simulink model "AC_FOC_PMSM_Developing_Rev_5_2022b"  (R2022b)
settings: Solver=VariableStepAuto  StartTime=0.0  StopTime=1  MaxStep=1e-4  RelTol=1e-3
values from neighbouring files (symbols this model uses):
  B = 11e-5    (= 0.00011)    [AB_FOC_For_PMSM_Parameters.m]
  Id_ref = 0    [AB_FOC_For_PMSM_Parameters.m]
  J = 0.47e-4    (= 4.7e-05)    [AB_FOC_For_PMSM_Parameters.m]
  Kcq = (2*zeta*wn*L) - Rs    (= 84.52)    [AB_FOC_For_PMSM_Parameters.m]
  Kcs = ((2*zeta*wns) - (B/J)) / ((1.5 *(pole^2)*flux)/J)    (= 0.00768666666667)    [AB_FOC_For_PMSM_Parameters.m]
  Ld = 7e-2    (= 0.07)    [AB_FOC_For_PMSM_Parameters.m]
  Lq = 7e-2    (= 0.07)    [AB_FOC_For_PMSM_Parameters.m]
  pole = 2    [AB_FOC_For_PMSM_Parameters.m]
  Rs = 2.98    [AB_FOC_For_PMSM_Parameters.m]
  speed_ref = 500    [AB_FOC_For_PMSM_Parameters.m]
libraries: fuzblock x10, slpidlib x9, spsDCVoltageSourceLib x5, spsPermanentMagnetSynchronousMachineLib x5, spsThreePhaseVIMeasurementLib x5, spsUniversalBridgeLib x5, spsdq0toabcLib x1, spspowerguiLib x1
(part 2 of 2)

== system AC_FOC_PMSM_Developing_Rev_5_2022b/FLC/Speed_Fuzzy_Control3 ==
  Speed_Motor : Inport
  Speed_Ref : Inport  Port=2
  Discrete PID Controller1 : slpidlib/PID Controller  Controller=I  Form=Parallel  TimeDomain=Discrete-time  UseExternalTs=off  SampleTime=-1  IntegratorMethod=Forward Euler  FilterMethod=Forward Euler  ControllerParametersSource=internal  P=1  I=0.5  UseKiTs=off  D=0  N=100  UseFilter=on  TunerSelectOption=Transfer Function Based (PID Tuner App)  InitialConditionSource=internal  InitialConditionForIntegrator=0  InitialConditionForFilter=0  DifferentiatorICPrevScaledInput=0  ExternalReset=none  TrackingMode=off  Kt=1  LimitOutput=off  SatLimitsSource=internal  UpperSaturationLimit=inf  LowerSaturationLimit=-inf  LinearizeAsGain=off  AntiWindupMode=none  Kb=1  LimitIntegrator=off  UpperIntegratorSaturationLimit=inf  LowerIntegratorSaturationLimit=-inf  POutMin=[]  POutMax=[]  IOutMin=[]  IOutMax=[]  DOutMin=[]  DOutMax=[]  NOutMin=[]  NOutMax=[]  SumOutMin=[]  SumOutMax=[]  SaturationOutMin=[]  SaturationOutMax=[]  PParamMin=[]  PParamMax=[]  IParamMin=[]  IParamMax=[]  DParamMin=[]  DParamMax=[]  NParamMin=[]  NParamMax=[]  KbParamMin=[]  KbParamMax=[]  KtParamMin=[]  KtParamMax=[]  KbOutMin=[]  KbOutMax=[]  KtOutMin=[]  KtOutMax=[]  IntegratorOutMin=[]  IntegratorOutMax=[]  FilterOutMin=[]  FilterOutMax=[]  SumI1OutMin=[]  SumI1OutMax=[]  SumI2OutMin=[]  SumI2OutMax=[]  SumI3OutMin=[]  SumI3OutMax=[]  SumI4OutMin=[]  SumI4OutMax=[]  SumDOutMin=[]  SumDOutMax=[]  DifferentiatorOutMin=[]  DifferentiatorOutMax=[]  FilterDiffOutCoefMin=[]  FilterDiffOutCoefMax=[]  ReciprocalOutMin=[]  ReciprocalOutMax=[]  SumDenOutMin=[]  SumDenOutMax=[]  SumNumOutMin=[]  SumNumOutMax=[]  DivideOutMin=[]  DivideOutMax=[]  UdiffTsProdOutMin=[]  UdiffTsProdOutMax=[]  NTsProdOutMin=[]  NTsProdOutMax=[]  UintegralTsProdOutMin=[]  UintegralTsProdOutMax=[]  UngainTsProdOutMin=[]  UngainTsProdOutMax=[]  IntegratorContinuousStateAttributes=''  IntegratorStateMustResolveToSignalObject=off  IntegratorRTWStateStorageClass=Auto  FilterContinuousStateAttributes=''  FilterStateMustResolveToSignalObject=off  FilterRTWStateStorageClass=Auto  ParallelPVariant=Disabled  IdealPVariant=Disabled  IVariant=InternalParameters  DVariant=Disabled  IntegratorVariant=Discrete  SatVariant=Disabled  AWVariant=Passthrough  PCopyVariant=Disabled  TRVariant=Disabled  FdbkBlocksVariant=Forward  IdealPFdbkVariant=Disabled  SatFdbkVariant=Disabled  DerivativeFilterVariant=Disabled  NVariant=Disabled  NCopyVariant=Disabled_SignalSpec  FilterICVariant=Disabled  IntegratorICVariant=InternalICs  ExternalResetVariant=Disabled  TRSumVariant=Passthrough  SumFdbkVariant=Disabled  SumVariant=Passthrough_I  TsampFilterVariant=InternalTs  TsampNgainVariant=Passthrough  TsampIntegralVariant=Disabled_SignalSpec  ExternalSaturationOutDataTypeStr=Inherit: Same as second input
      settings: LibrarySourceBlock=simulink/Discrete/Discrete PID Controller
  Fuzzy Logic Controller : fuzblock/Fuzzy Logic  Controller  FIS='FOC_PMSM_25_Test.fis'  OutputSampleNumber=101  DataType=double  FuzzifiedInputs=off  RuleFiringStrengths=off  RuleOutputs=off  AggregatedOutputs=off  SimulateUsing=Interpreted execution  OutOfRangeInputValueMessage=warning  NoRuleFiredMessage=warning  EmptyOutputFuzzySetMessage=warning
  Mux6 : Mux  Inputs=2
  Scope : Scope  NumInputPorts=4
  Scope1 : Scope
  Sum5 : Sum  Inputs=|+-
  Unit Delay : UnitDelay  SampleTime=-1  HasFrameUpgradeWarning=on
  Zero-Order Hold : ZeroOrderHold  SampleTime=-1
  Speed_Control : Outport
  wires:
  Mux6/1 -> Fuzzy Logic Controller/1
  Zero-Order Hold/1 -> Mux6/1, Unit Delay/1, Scope/3
  Unit Delay/1 -> Mux6/2, Scope1/1
  Speed_Motor/1 -> Scope/2, Sum5/2
  Speed_Ref/1 -> Scope/1, Sum5/1
  Fuzzy Logic Controller/1 -> Speed_Control/1
  Sum5/1 -> Zero-Order Hold/1

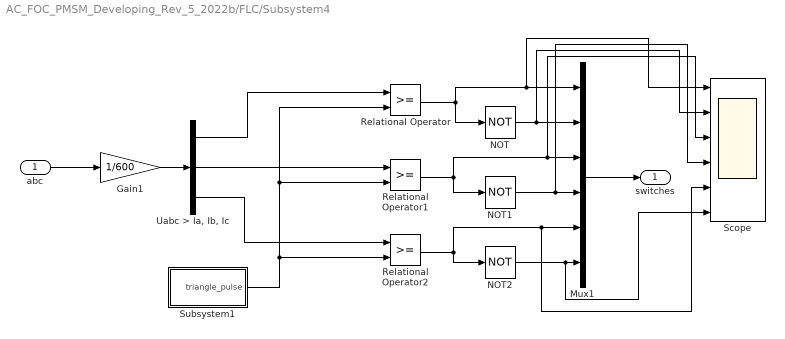
== system AC_FOC_PMSM_Developing_Rev_5_2022b/FLC/Subsystem4 ==
  abc : Inport
  Gain1 : Gain  Gain=1/600
  Mux1 : Mux  Inputs=6
  NOT : Logic  Operator=NOT  IconShape=distinctive  AllPortsSameDT=off  OutDataTypeStr=boolean
  NOT1 : Logic  Operator=NOT  IconShape=distinctive  AllPortsSameDT=off  OutDataTypeStr=boolean
  NOT2 : Logic  Operator=NOT  IconShape=distinctive  AllPortsSameDT=off  OutDataTypeStr=boolean
  Relational Operator : RelationalOperator  OutDataTypeStr=boolean  RndMeth=Simplest  InputSameDT=off
  Relational Operator1 : RelationalOperator  OutDataTypeStr=boolean  RndMeth=Simplest  InputSameDT=off
  Relational Operator2 : RelationalOperator  OutDataTypeStr=boolean  RndMeth=Simplest  InputSameDT=off
  Scope : Scope  NumInputPorts=6
  Subsystem1 : Subsystem
  "Uabc > Ia, Ib, Ic" : Demux  Outputs=3
  switches : Outport
  wires:
  NOT/1 -> Scope/2, Mux1/2
  NOT1/1 -> Scope/4, Mux1/4
  "Uabc > Ia, Ib, Ic"/2 -> Relational Operator1/1
  Gain1/1 -> "Uabc > Ia, Ib, Ic"/1
  "Uabc > Ia, Ib, Ic"/1 -> Relational Operator/1
  NOT2/1 -> Scope/6, Mux1/6
  Relational Operator1/1 -> Scope/3, Mux1/3, NOT1/1
  "Uabc > Ia, Ib, Ic"/3 -> Relational Operator2/1
  abc/1 -> Gain1/1
  Mux1/1 -> switches/1
  Relational Operator/1 -> NOT/1, Scope/1, Mux1/1
  Relational Operator2/1 -> Scope/5, Mux1/5, NOT2/1
  Subsystem1/1(triangle_pulse) -> Relational Operator/2, Relational Operator1/2, Relational Operator2/2

== system AC_FOC_PMSM_Developing_Rev_5_2022b/PID/Clark_Park Transformation ==
  Ia : Inport
  Ib : Inport  Port=2
  Ic : Inport  Port=3
  Theta : Inport  Port=4
  Gain : Gain  Gain=2/3
  Gain2 : Gain  Gain=-2/3
  Mux : Mux
  "iabc -> id" : Fcn  Expr=u(1) * sin(u(4)) + u(2) *sin(u(4) - 2*pi/3) + u(3)*sin(u(4)+2*pi/3)
  "iabc -> iq" : Fcn  Expr=u(1) * cos(u(4)) + u(2) *cos(u(4) - 2*pi/3) + u(3)*cos(u(4)+2*pi/3)
  iq : Outport
  id : Outport  Port=2
  wires:
  Gain2/1 -> id/1  "id"
  Gain/1 -> iq/1  "iq"
  "iabc -> id"/1 -> Gain2/1
  "iabc -> iq"/1 -> Gain/1
  Mux/1 -> "iabc -> iq"/1, "iabc -> id"/1
  Ia/1 -> Mux/1
  Ib/1 -> Mux/2
  Ic/1 -> Mux/3
  Theta/1 -> Mux/4

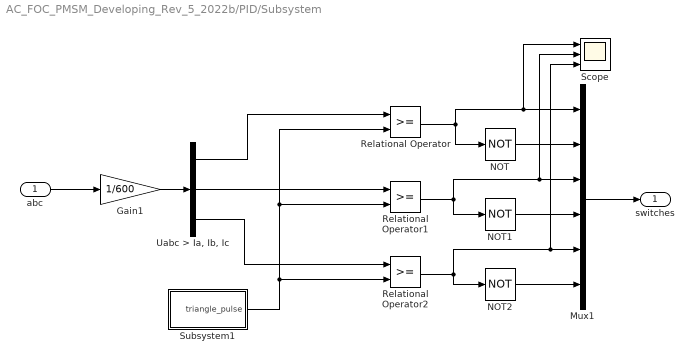
== system AC_FOC_PMSM_Developing_Rev_5_2022b/PID/Subsystem ==
  abc : Inport
  Gain1 : Gain  Gain=1/600
  Mux1 : Mux  Inputs=6
  NOT : Logic  Operator=NOT  IconShape=distinctive  AllPortsSameDT=off  OutDataTypeStr=boolean
  NOT1 : Logic  Operator=NOT  IconShape=distinctive  AllPortsSameDT=off  OutDataTypeStr=boolean
  NOT2 : Logic  Operator=NOT  IconShape=distinctive  AllPortsSameDT=off  OutDataTypeStr=boolean
  Relational Operator : RelationalOperator  OutDataTypeStr=boolean  RndMeth=Simplest  InputSameDT=off
  Relational Operator1 : RelationalOperator  OutDataTypeStr=boolean  RndMeth=Simplest  InputSameDT=off
  Relational Operator2 : RelationalOperator  OutDataTypeStr=boolean  RndMeth=Simplest  InputSameDT=off
  Scope : Scope  NumInputPorts=3
  Subsystem1 : Subsystem
  "Uabc > Ia, Ib, Ic" : Demux  Outputs=3
  switches : Outport
  wires:
  NOT/1 -> Mux1/2
  NOT1/1 -> Mux1/4
  "Uabc > Ia, Ib, Ic"/2 -> Relational Operator1/1
  Gain1/1 -> "Uabc > Ia, Ib, Ic"/1
  "Uabc > Ia, Ib, Ic"/1 -> Relational Operator/1
  NOT2/1 -> Mux1/6
  Relational Operator1/1 -> Scope/2, Mux1/3, NOT1/1
  "Uabc > Ia, Ib, Ic"/3 -> Relational Operator2/1
  abc/1 -> Gain1/1
  Mux1/1 -> switches/1
  Relational Operator/1 -> NOT/1, Scope/1, Mux1/1
  Relational Operator2/1 -> Scope/3, Mux1/5, NOT2/1
  Subsystem1/1(triangle_pulse) -> Relational Operator/2, Relational Operator1/2, Relational Operator2/2

== system AC_FOC_PMSM_Developing_Rev_5_2022b/Simplified_FLC/Clark_Park Transformation4 ==
  Ia : Inport
  Ib : Inport  Port=2
  Ic : Inport  Port=3
  Theta : Inport  Port=4
  Gain : Gain  Gain=2/3
  Gain2 : Gain  Gain=-2/3
  Mux : Mux
  "iabc -> id" : Fcn  Expr=u(1) * sin(u(4)) + u(2) *sin(u(4) - 2*pi/3) + u(3)*sin(u(4)+2*pi/3)
  "iabc -> iq" : Fcn  Expr=u(1) * cos(u(4)) + u(2) *cos(u(4) - 2*pi/3) + u(3)*cos(u(4)+2*pi/3)
  iq : Outport
  id : Outport  Port=2
  wires:
  Gain2/1 -> id/1  "id"
  Gain/1 -> iq/1  "iq"
  "iabc -> id"/1 -> Gain2/1
  "iabc -> iq"/1 -> Gain/1
  Mux/1 -> "iabc -> iq"/1, "iabc -> id"/1
  Ia/1 -> Mux/1
  Ib/1 -> Mux/2
  Ic/1 -> Mux/3
  Theta/1 -> Mux/4

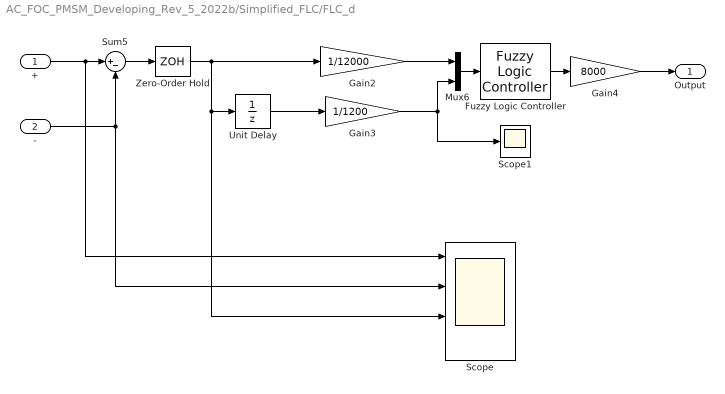
== system AC_FOC_PMSM_Developing_Rev_5_2022b/Simplified_FLC/FLC_d ==
  + : Inport
  - : Inport  Port=2
  Fuzzy Logic Controller : fuzblock/Fuzzy Logic  Controller  FIS='FOC_PMSM_25_Simplified.fis'  OutputSampleNumber=101  DataType=double  FuzzifiedInputs=off  RuleFiringStrengths=off  RuleOutputs=off  AggregatedOutputs=off  SimulateUsing=Interpreted execution  OutOfRangeInputValueMessage=warning  NoRuleFiredMessage=warning  EmptyOutputFuzzySetMessage=warning
  Gain2 : Gain  Gain=1/12000
  Gain3 : Gain  Gain=1/1200
  Gain4 : Gain  Gain=8000
  Mux6 : Mux  Inputs=2
  Scope : Scope  NumInputPorts=4
  Scope1 : Scope
  Sum5 : Sum  Inputs=|+-
  Unit Delay : UnitDelay  SampleTime=-1  HasFrameUpgradeWarning=on
  Zero-Order Hold : ZeroOrderHold  SampleTime=-1
  Output : Outport
  wires:
  Fuzzy Logic Controller/1 -> Gain4/1
  Mux6/1 -> Fuzzy Logic Controller/1
  Gain2/1 -> Mux6/1
  Gain3/1 -> Scope1/1, Mux6/2
  Gain4/1 -> Output/1
  Sum5/1 -> Zero-Order Hold/1
  -/1 -> Scope/2, Sum5/2
  +/1 -> Scope/1, Sum5/1
  Zero-Order Hold/1 -> Gain2/1, Scope/3, Unit Delay/1
  Unit Delay/1 -> Gain3/1

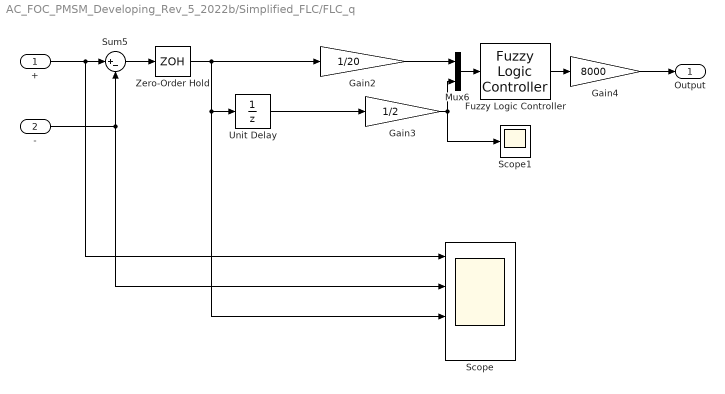
== system AC_FOC_PMSM_Developing_Rev_5_2022b/Simplified_FLC/FLC_q ==
  + : Inport
  - : Inport  Port=2
  Fuzzy Logic Controller : fuzblock/Fuzzy Logic  Controller  FIS='FOC_PMSM_25_Simplified.fis'  OutputSampleNumber=101  DataType=double  FuzzifiedInputs=off  RuleFiringStrengths=off  RuleOutputs=off  AggregatedOutputs=off  SimulateUsing=Interpreted execution  OutOfRangeInputValueMessage=warning  NoRuleFiredMessage=warning  EmptyOutputFuzzySetMessage=warning
  Gain2 : Gain  Gain=1/20
  Gain3 : Gain  Gain=1/2
  Gain4 : Gain  Gain=8000
  Mux6 : Mux  Inputs=2
  Scope : Scope  NumInputPorts=4
  Scope1 : Scope
  Sum5 : Sum  Inputs=|+-
  Unit Delay : UnitDelay  SampleTime=-1  HasFrameUpgradeWarning=on
  Zero-Order Hold : ZeroOrderHold  SampleTime=-1
  Output : Outport
  wires:
  Fuzzy Logic Controller/1 -> Gain4/1
  Mux6/1 -> Fuzzy Logic Controller/1
  Gain2/1 -> Mux6/1
  Gain3/1 -> Mux6/2, Scope1/1
  Gain4/1 -> Output/1
  Sum5/1 -> Zero-Order Hold/1
  -/1 -> Scope/2, Sum5/2
  +/1 -> Scope/1, Sum5/1
  Zero-Order Hold/1 -> Gain2/1, Scope/3, Unit Delay/1
  Unit Delay/1 -> Gain3/1

== system AC_FOC_PMSM_Developing_Rev_5_2022b/Simplified_FLC/Inverse Park-Clarke3 ==
  Iq : Inport
  Id : Inport  Port=2
  theta : Inport  Port=3
  Inverse Clarke : Subsystem
  Inverse Park : Subsystem
  Mux3 : Mux  Inputs=3
  abc : Outport
  wires:
  Inverse Park/1(alpha) -> Inverse Clarke/1(alpha)
  Inverse Clarke/2(b) -> Mux3/2
  Inverse Park/2(beta) -> Inverse Clarke/2(beta)
  Mux3/1 -> abc/1
  Inverse Clarke/1(a) -> Mux3/1
  theta/1 -> Inverse Park/3(theta)
  Iq/1 -> Inverse Park/2(Iq)
  Inverse Clarke/3(c) -> Mux3/3
  Id/1 -> Inverse Park/1(Id)

== system AC_FOC_PMSM_Developing_Rev_5_2022b/Simplified_FLC/Speed_Fuzzy_Control3 ==
  Speed_Motor : Inport
  Speed_Ref : Inport  Port=2
  Fuzzy Logic Controller : fuzblock/Fuzzy Logic  Controller  FIS='FOC_PMSM_25_Simplified.fis'  OutputSampleNumber=101  DataType=double  FuzzifiedInputs=off  RuleFiringStrengths=off  RuleOutputs=off  AggregatedOutputs=off  SimulateUsing=Interpreted execution  OutOfRangeInputValueMessage=warning  NoRuleFiredMessage=warning  EmptyOutputFuzzySetMessage=warning
  Gain2 : Gain  Gain=1/2500
  Gain3 : Gain  Gain=1/2500
  Gain4 : Gain  Gain=50
  Mux6 : Mux  Inputs=2
  Scope : Scope  NumInputPorts=4
  Scope1 : Scope
  Sum5 : Sum  Inputs=|+-
  Unit Delay : UnitDelay  SampleTime=-1  HasFrameUpgradeWarning=on
  Zero-Order Hold : ZeroOrderHold  SampleTime=-1
  Speed_Control : Outport
  wires:
  Fuzzy Logic Controller/1 -> Gain4/1
  Mux6/1 -> Fuzzy Logic Controller/1
  Gain2/1 -> Mux6/1
  Gain3/1 -> Mux6/2, Scope1/1
  Gain4/1 -> Speed_Control/1
  Sum5/1 -> Zero-Order Hold/1
  Speed_Motor/1 -> Scope/2, Sum5/2
  Speed_Ref/1 -> Scope/1, Sum5/1
  Zero-Order Hold/1 -> Gain2/1, Unit Delay/1, Scope/3
  Unit Delay/1 -> Gain3/1

== system AC_FOC_PMSM_Developing_Rev_5_2022b/Simplified_FLC/Subsystem4 ==
  abc : Inport
  Gain1 : Gain  Gain=1/600
  Mux1 : Mux  Inputs=6
  NOT : Logic  Operator=NOT  IconShape=distinctive  AllPortsSameDT=off  OutDataTypeStr=boolean
  NOT1 : Logic  Operator=NOT  IconShape=distinctive  AllPortsSameDT=off  OutDataTypeStr=boolean
  NOT2 : Logic  Operator=NOT  IconShape=distinctive  AllPortsSameDT=off  OutDataTypeStr=boolean
  Relational Operator : RelationalOperator  OutDataTypeStr=boolean  RndMeth=Simplest  InputSameDT=off
  Relational Operator1 : RelationalOperator  OutDataTypeStr=boolean  RndMeth=Simplest  InputSameDT=off
  Relational Operator2 : RelationalOperator  OutDataTypeStr=boolean  RndMeth=Simplest  InputSameDT=off
  Scope : Scope  NumInputPorts=6
  Subsystem1 : Subsystem
  "Uabc > Ia, Ib, Ic" : Demux  Outputs=3
  switches : Outport
  wires:
  NOT/1 -> Scope/2, Mux1/2
  NOT1/1 -> Scope/4, Mux1/4
  "Uabc > Ia, Ib, Ic"/2 -> Relational Operator1/1
  Gain1/1 -> "Uabc > Ia, Ib, Ic"/1
  "Uabc > Ia, Ib, Ic"/1 -> Relational Operator/1
  NOT2/1 -> Scope/6, Mux1/6
  Relational Operator1/1 -> Scope/3, Mux1/3, NOT1/1
  "Uabc > Ia, Ib, Ic"/3 -> Relational Operator2/1
  abc/1 -> Gain1/1
  Mux1/1 -> switches/1
  Relational Operator/1 -> NOT/1, Scope/1, Mux1/1
  Relational Operator2/1 -> Scope/5, Mux1/5, NOT2/1
  Subsystem1/1(triangle_pulse) -> Relational Operator/2, Relational Operator1/2, Relational Operator2/2

== system AC_FOC_PMSM_Developing_Rev_5_2022b/Simplified_Speed_Q_FLC_D_PID1/Clark_Park Transformation4 ==
  Ia : Inport
  Ib : Inport  Port=2
  Ic : Inport  Port=3
  Theta : Inport  Port=4
  Gain : Gain  Gain=2/3
  Gain2 : Gain  Gain=-2/3
  Mux : Mux
  "iabc -> id" : Fcn  Expr=u(1) * sin(u(4)) + u(2) *sin(u(4) - 2*pi/3) + u(3)*sin(u(4)+2*pi/3)
  "iabc -> iq" : Fcn  Expr=u(1) * cos(u(4)) + u(2) *cos(u(4) - 2*pi/3) + u(3)*cos(u(4)+2*pi/3)
  iq : Outport
  id : Outport  Port=2
  wires:
  Gain2/1 -> id/1  "id"
  Gain/1 -> iq/1  "iq"
  "iabc -> id"/1 -> Gain2/1
  "iabc -> iq"/1 -> Gain/1
  Mux/1 -> "iabc -> iq"/1, "iabc -> id"/1
  Ia/1 -> Mux/1
  Ib/1 -> Mux/2
  Ic/1 -> Mux/3
  Theta/1 -> Mux/4

== system AC_FOC_PMSM_Developing_Rev_5_2022b/Simplified_Speed_Q_FLC_D_PID1/FLC_q2 ==
  + : Inport
  - : Inport  Port=2
  Fuzzy Logic Controller : fuzblock/Fuzzy Logic  Controller  FIS='FOC_PMSM_25.fis'  OutputSampleNumber=101  DataType=double  FuzzifiedInputs=off  RuleFiringStrengths=off  RuleOutputs=off  AggregatedOutputs=off  SimulateUsing=Interpreted execution  OutOfRangeInputValueMessage=warning  NoRuleFiredMessage=warning  EmptyOutputFuzzySetMessage=warning
  Gain2 : Gain  Gain=1/20
  Gain3 : Gain  Gain=1/2
  Gain4 : Gain  Gain=8000
  Mux6 : Mux  Inputs=2
  Scope : Scope  NumInputPorts=4
  Scope1 : Scope
  Sum5 : Sum  Inputs=|+-
  Unit Delay : UnitDelay  SampleTime=-1  HasFrameUpgradeWarning=on
  Zero-Order Hold : ZeroOrderHold  SampleTime=-1
  Output : Outport
  wires:
  Fuzzy Logic Controller/1 -> Gain4/1
  Mux6/1 -> Fuzzy Logic Controller/1
  Gain2/1 -> Mux6/1
  Gain3/1 -> Mux6/2, Scope1/1
  Gain4/1 -> Output/1
  Sum5/1 -> Zero-Order Hold/1
  -/1 -> Scope/2, Sum5/2
  +/1 -> Scope/1, Sum5/1
  Zero-Order Hold/1 -> Gain2/1, Scope/3, Unit Delay/1
  Unit Delay/1 -> Gain3/1

== system AC_FOC_PMSM_Developing_Rev_5_2022b/Simplified_Speed_Q_FLC_D_PID1/Inverse Park-Clarke3 ==
  Iq : Inport
  Id : Inport  Port=2
  theta : Inport  Port=3
  Inverse Clarke : Subsystem
  Inverse Park : Subsystem
  Mux3 : Mux  Inputs=3
  abc : Outport
  wires:
  Inverse Park/1(alpha) -> Inverse Clarke/1(alpha)
  Inverse Clarke/2(b) -> Mux3/2
  Inverse Park/2(beta) -> Inverse Clarke/2(beta)
  Mux3/1 -> abc/1
  Inverse Clarke/1(a) -> Mux3/1
  theta/1 -> Inverse Park/3(theta)
  Iq/1 -> Inverse Park/2(Iq)
  Inverse Clarke/3(c) -> Mux3/3
  Id/1 -> Inverse Park/1(Id)

== system AC_FOC_PMSM_Developing_Rev_5_2022b/Simplified_Speed_Q_FLC_D_PID1/Speed_Fuzzy_Control3 ==
  Speed_Motor : Inport
  Speed_Ref : Inport  Port=2
  Fuzzy Logic Controller : fuzblock/Fuzzy Logic  Controller  FIS='FOC_PMSM_25_Simplified.fis'  OutputSampleNumber=101  DataType=double  FuzzifiedInputs=off  RuleFiringStrengths=off  RuleOutputs=off  AggregatedOutputs=off  SimulateUsing=Interpreted execution  OutOfRangeInputValueMessage=warning  NoRuleFiredMessage=warning  EmptyOutputFuzzySetMessage=warning
  Gain2 : Gain  Gain=1/2500
  Gain3 : Gain  Gain=1/2500
  Gain4 : Gain  Gain=50
  Mux6 : Mux  Inputs=2
  Scope : Scope  NumInputPorts=4
  Scope1 : Scope
  Sum5 : Sum  Inputs=|+-
  Unit Delay : UnitDelay  SampleTime=-1  HasFrameUpgradeWarning=on
  Zero-Order Hold : ZeroOrderHold  SampleTime=-1
  Speed_Control : Outport
  wires:
  Fuzzy Logic Controller/1 -> Gain4/1
  Mux6/1 -> Fuzzy Logic Controller/1
  Gain2/1 -> Mux6/1
  Gain3/1 -> Mux6/2, Scope1/1
  Gain4/1 -> Speed_Control/1
  Sum5/1 -> Zero-Order Hold/1
  Speed_Motor/1 -> Scope/2, Sum5/2
  Speed_Ref/1 -> Scope/1, Sum5/1
  Zero-Order Hold/1 -> Gain2/1, Unit Delay/1, Scope/3
  Unit Delay/1 -> Gain3/1

== system AC_FOC_PMSM_Developing_Rev_5_2022b/Simplified_Speed_Q_FLC_D_PID1/Subsystem4 ==
  abc : Inport
  Gain1 : Gain  Gain=1/600
  Mux1 : Mux  Inputs=6
  NOT : Logic  Operator=NOT  IconShape=distinctive  AllPortsSameDT=off  OutDataTypeStr=boolean
  NOT1 : Logic  Operator=NOT  IconShape=distinctive  AllPortsSameDT=off  OutDataTypeStr=boolean
  NOT2 : Logic  Operator=NOT  IconShape=distinctive  AllPortsSameDT=off  OutDataTypeStr=boolean
  Relational Operator : RelationalOperator  OutDataTypeStr=boolean  RndMeth=Simplest  InputSameDT=off
  Relational Operator1 : RelationalOperator  OutDataTypeStr=boolean  RndMeth=Simplest  InputSameDT=off
  Relational Operator2 : RelationalOperator  OutDataTypeStr=boolean  RndMeth=Simplest  InputSameDT=off
  Scope : Scope  NumInputPorts=6
  Subsystem1 : Subsystem
  "Uabc > Ia, Ib, Ic" : Demux  Outputs=3
  switches : Outport
  wires:
  NOT/1 -> Scope/2, Mux1/2
  NOT1/1 -> Scope/4, Mux1/4
  "Uabc > Ia, Ib, Ic"/2 -> Relational Operator1/1
  Gain1/1 -> "Uabc > Ia, Ib, Ic"/1
  "Uabc > Ia, Ib, Ic"/1 -> Relational Operator/1
  NOT2/1 -> Scope/6, Mux1/6
  Relational Operator1/1 -> Scope/3, Mux1/3, NOT1/1
  "Uabc > Ia, Ib, Ic"/3 -> Relational Operator2/1
  abc/1 -> Gain1/1
  Mux1/1 -> switches/1
  Relational Operator/1 -> NOT/1, Scope/1, Mux1/1
  Relational Operator2/1 -> Scope/5, Mux1/5, NOT2/1
  Subsystem1/1(triangle_pulse) -> Relational Operator/2, Relational Operator1/2, Relational Operator2/2

== system AC_FOC_PMSM_Developing_Rev_5_2022b/Speed_Q_FLC_D_PID/Clark_Park Transformation4 ==
  Ia : Inport
  Ib : Inport  Port=2
  Ic : Inport  Port=3
  Theta : Inport  Port=4
  Gain : Gain  Gain=2/3
  Gain2 : Gain  Gain=-2/3
  Mux : Mux
  "iabc -> id" : Fcn  Expr=u(1) * sin(u(4)) + u(2) *sin(u(4) - 2*pi/3) + u(3)*sin(u(4)+2*pi/3)
  "iabc -> iq" : Fcn  Expr=u(1) * cos(u(4)) + u(2) *cos(u(4) - 2*pi/3) + u(3)*cos(u(4)+2*pi/3)
  iq : Outport
  id : Outport  Port=2
  wires:
  Gain2/1 -> id/1  "id"
  Gain/1 -> iq/1  "iq"
  "iabc -> id"/1 -> Gain2/1
  "iabc -> iq"/1 -> Gain/1
  Mux/1 -> "iabc -> iq"/1, "iabc -> id"/1
  Ia/1 -> Mux/1
  Ib/1 -> Mux/2
  Ic/1 -> Mux/3
  Theta/1 -> Mux/4

== system AC_FOC_PMSM_Developing_Rev_5_2022b/Speed_Q_FLC_D_PID/FLC_q2 ==
  + : Inport
  - : Inport  Port=2
  Fuzzy Logic Controller : fuzblock/Fuzzy Logic  Controller  FIS='FOC_PMSM_25.fis'  OutputSampleNumber=101  DataType=double  FuzzifiedInputs=off  RuleFiringStrengths=off  RuleOutputs=off  AggregatedOutputs=off  SimulateUsing=Interpreted execution  OutOfRangeInputValueMessage=warning  NoRuleFiredMessage=warning  EmptyOutputFuzzySetMessage=warning
  Gain2 : Gain  Gain=1/20
  Gain3 : Gain  Gain=1/2
  Gain4 : Gain  Gain=8000
  Mux6 : Mux  Inputs=2
  Scope : Scope  NumInputPorts=4
  Scope1 : Scope
  Sum5 : Sum  Inputs=|+-
  Unit Delay : UnitDelay  SampleTime=-1  HasFrameUpgradeWarning=on
  Zero-Order Hold : ZeroOrderHold  SampleTime=-1
  Output : Outport
  wires:
  Fuzzy Logic Controller/1 -> Gain4/1
  Mux6/1 -> Fuzzy Logic Controller/1
  Gain2/1 -> Mux6/1
  Gain3/1 -> Mux6/2, Scope1/1
  Gain4/1 -> Output/1
  Sum5/1 -> Zero-Order Hold/1
  -/1 -> Scope/2, Sum5/2
  +/1 -> Scope/1, Sum5/1
  Zero-Order Hold/1 -> Gain2/1, Scope/3, Unit Delay/1
  Unit Delay/1 -> Gain3/1

== system AC_FOC_PMSM_Developing_Rev_5_2022b/Speed_Q_FLC_D_PID/Inverse Park-Clarke3 ==
  Iq : Inport
  Id : Inport  Port=2
  theta : Inport  Port=3
  Inverse Clarke : Subsystem
  Inverse Park : Subsystem
  Mux3 : Mux  Inputs=3
  abc : Outport
  wires:
  Inverse Park/1(alpha) -> Inverse Clarke/1(alpha)
  Inverse Clarke/2(b) -> Mux3/2
  Inverse Park/2(beta) -> Inverse Clarke/2(beta)
  Mux3/1 -> abc/1
  Inverse Clarke/1(a) -> Mux3/1
  theta/1 -> Inverse Park/3(theta)
  Iq/1 -> Inverse Park/2(Iq)
  Inverse Clarke/3(c) -> Mux3/3
  Id/1 -> Inverse Park/1(Id)

== system AC_FOC_PMSM_Developing_Rev_5_2022b/Speed_Q_FLC_D_PID/Speed_Fuzzy_Control3 ==
  Speed_Motor : Inport
  Speed_Ref : Inport  Port=2
  Fuzzy Logic Controller : fuzblock/Fuzzy Logic  Controller  FIS='FOC_PMSM_25.fis'  OutputSampleNumber=101  DataType=double  FuzzifiedInputs=off  RuleFiringStrengths=off  RuleOutputs=off  AggregatedOutputs=off  SimulateUsing=Interpreted execution  OutOfRangeInputValueMessage=warning  NoRuleFiredMessage=warning  EmptyOutputFuzzySetMessage=warning
  Gain2 : Gain  Gain=1/2500
  Gain3 : Gain  Gain=1/2500
  Gain4 : Gain  Gain=50
  Mux6 : Mux  Inputs=2
  Scope : Scope  NumInputPorts=4
  Scope1 : Scope
  Sum5 : Sum  Inputs=|+-
  Unit Delay : UnitDelay  SampleTime=-1  HasFrameUpgradeWarning=on
  Zero-Order Hold : ZeroOrderHold  SampleTime=-1
  Speed_Control : Outport
  wires:
  Fuzzy Logic Controller/1 -> Gain4/1
  Mux6/1 -> Fuzzy Logic Controller/1
  Gain2/1 -> Mux6/1
  Gain3/1 -> Mux6/2, Scope1/1
  Gain4/1 -> Speed_Control/1
  Sum5/1 -> Zero-Order Hold/1
  Speed_Motor/1 -> Scope/2, Sum5/2
  Speed_Ref/1 -> Scope/1, Sum5/1
  Zero-Order Hold/1 -> Gain2/1, Unit Delay/1, Scope/3
  Unit Delay/1 -> Gain3/1

== system AC_FOC_PMSM_Developing_Rev_5_2022b/Speed_Q_FLC_D_PID/Subsystem4 ==
  abc : Inport
  Gain1 : Gain  Gain=1/600
  Mux1 : Mux  Inputs=6
  NOT : Logic  Operator=NOT  IconShape=distinctive  AllPortsSameDT=off  OutDataTypeStr=boolean
  NOT1 : Logic  Operator=NOT  IconShape=distinctive  AllPortsSameDT=off  OutDataTypeStr=boolean
  NOT2 : Logic  Operator=NOT  IconShape=distinctive  AllPortsSameDT=off  OutDataTypeStr=boolean
  Relational Operator : RelationalOperator  OutDataTypeStr=boolean  RndMeth=Simplest  InputSameDT=off
  Relational Operator1 : RelationalOperator  OutDataTypeStr=boolean  RndMeth=Simplest  InputSameDT=off
  Relational Operator2 : RelationalOperator  OutDataTypeStr=boolean  RndMeth=Simplest  InputSameDT=off
  Scope : Scope  NumInputPorts=6
  Subsystem1 : Subsystem
  "Uabc > Ia, Ib, Ic" : Demux  Outputs=3
  switches : Outport
  wires:
  NOT/1 -> Scope/2, Mux1/2
  NOT1/1 -> Scope/4, Mux1/4
  "Uabc > Ia, Ib, Ic"/2 -> Relational Operator1/1
  Gain1/1 -> "Uabc > Ia, Ib, Ic"/1
  "Uabc > Ia, Ib, Ic"/1 -> Relational Operator/1
  NOT2/1 -> Scope/6, Mux1/6
  Relational Operator1/1 -> Scope/3, Mux1/3, NOT1/1
  "Uabc > Ia, Ib, Ic"/3 -> Relational Operator2/1
  abc/1 -> Gain1/1
  Mux1/1 -> switches/1
  Relational Operator/1 -> NOT/1, Scope/1, Mux1/1
  Relational Operator2/1 -> Scope/5, Mux1/5, NOT2/1
  Subsystem1/1(triangle_pulse) -> Relational Operator/2, Relational Operator1/2, Relational Operator2/2

== system AC_FOC_PMSM_Developing_Rev_5_2022b/FLC/Inverse Park-Clarke3/Inverse Clarke ==
  alpha : Inport
  beta : Inport  Port=2
  "    " : Fcn  Expr=-u(1)/2 + u(2)*sqrt(3)/2
  "        " : Fcn  Expr=-u(1)/2 - u(2)*sqrt(3)/2
  Mux3 : Mux  Inputs=2
  a : Outport
  b : Outport  Port=2
  c : Outport  Port=3
  wires:
  alpha/1 -> a/1, Mux3/1
  beta/1 -> Mux3/2
  Mux3/1 -> "    "/1, "        "/1
  "        "/1 -> c/1
  "    "/1 -> b/1

== system AC_FOC_PMSM_Developing_Rev_5_2022b/FLC/Inverse Park-Clarke3/Inverse Park ==
  Id : Inport
  Iq : Inport  Port=2
  theta : Inport  Port=3
  " " : Fcn  Expr=cos(u(3))*u(1)-sin(u(3))*u(2)
  "  " : Fcn  Expr=sin(u(3))*u(1)+cos(u(3))*u(2)
  Mux : Mux  Inputs=3
  alpha : Outport
  beta : Outport  Port=2
  wires:
  Mux/1 -> " "/1, "  "/1
  theta/1 -> Mux/3
  Id/1 -> Mux/1
  Iq/1 -> Mux/2
  " "/1 -> alpha/1
  "  "/1 -> beta/1

== system AC_FOC_PMSM_Developing_Rev_5_2022b/FLC/Subsystem4/Subsystem1 ==
  Constant : Constant
  Constant1 : Constant
  Gain : Gain  Gain=2*10000
  Gain1 : Gain  Gain=2
  Integrator : Integrator
  Pulse Generator : DiscretePulseGenerator  PulseType=Time based  Amplitude=2  Period=1/10000  PulseWidth=50
  Sum3 : Sum  Inputs=|+-
  Sum4 : Sum  Inputs=|+-
  triangle_pulse : Outport
  wires:
  Integrator/1 -> Gain/1
  Sum4/1 -> triangle_pulse/1
  Sum3/1 -> Integrator/1
  Gain/1 -> Gain1/1
  Constant1/1 -> Sum4/2
  Constant/1 -> Sum3/2
  Gain1/1 -> Sum4/1
  Pulse Generator/1 -> Sum3/1

== system AC_FOC_PMSM_Developing_Rev_5_2022b/PID/Subsystem/Subsystem1 ==
  Constant : Constant
  Constant1 : Constant
  Gain : Gain  Gain=2*10000
  Gain1 : Gain  Gain=2
  Integrator : Integrator
  Pulse Generator : DiscretePulseGenerator  PulseType=Time based  Amplitude=2  Period=1/10000  PulseWidth=50
  Sum3 : Sum  Inputs=|+-
  Sum4 : Sum  Inputs=|+-
  triangle_pulse : Outport
  wires:
  Integrator/1 -> Gain/1
  Sum4/1 -> triangle_pulse/1
  Sum3/1 -> Integrator/1
  Gain/1 -> Gain1/1
  Constant1/1 -> Sum4/2
  Constant/1 -> Sum3/2
  Gain1/1 -> Sum4/1
  Pulse Generator/1 -> Sum3/1

== system AC_FOC_PMSM_Developing_Rev_5_2022b/Simplified_FLC/Inverse Park-Clarke3/Inverse Clarke ==
  alpha : Inport
  beta : Inport  Port=2
  "    " : Fcn  Expr=-u(1)/2 + u(2)*sqrt(3)/2
  "        " : Fcn  Expr=-u(1)/2 - u(2)*sqrt(3)/2
  Mux3 : Mux  Inputs=2
  a : Outport
  b : Outport  Port=2
  c : Outport  Port=3
  wires:
  alpha/1 -> a/1, Mux3/1
  beta/1 -> Mux3/2
  Mux3/1 -> "    "/1, "        "/1
  "        "/1 -> c/1
  "    "/1 -> b/1

== system AC_FOC_PMSM_Developing_Rev_5_2022b/Simplified_FLC/Inverse Park-Clarke3/Inverse Park ==
  Id : Inport
  Iq : Inport  Port=2
  theta : Inport  Port=3
  " " : Fcn  Expr=cos(u(3))*u(1)-sin(u(3))*u(2)
  "  " : Fcn  Expr=sin(u(3))*u(1)+cos(u(3))*u(2)
  Mux : Mux  Inputs=3
  alpha : Outport
  beta : Outport  Port=2
  wires:
  Mux/1 -> " "/1, "  "/1
  theta/1 -> Mux/3
  Id/1 -> Mux/1
  Iq/1 -> Mux/2
  " "/1 -> alpha/1
  "  "/1 -> beta/1

== system AC_FOC_PMSM_Developing_Rev_5_2022b/Simplified_FLC/Subsystem4/Subsystem1 ==
  Constant : Constant
  Constant1 : Constant
  Gain : Gain  Gain=2*10000
  Gain1 : Gain  Gain=2
  Integrator : Integrator
  Pulse Generator : DiscretePulseGenerator  PulseType=Time based  Amplitude=2  Period=1/10000  PulseWidth=50
  Sum3 : Sum  Inputs=|+-
  Sum4 : Sum  Inputs=|+-
  triangle_pulse : Outport
  wires:
  Integrator/1 -> Gain/1
  Sum4/1 -> triangle_pulse/1
  Sum3/1 -> Integrator/1
  Gain/1 -> Gain1/1
  Constant1/1 -> Sum4/2
  Constant/1 -> Sum3/2
  Gain1/1 -> Sum4/1
  Pulse Generator/1 -> Sum3/1

== system AC_FOC_PMSM_Developing_Rev_5_2022b/Simplified_Speed_Q_FLC_D_PID1/Inverse Park-Clarke3/Inverse Clarke ==
  alpha : Inport
  beta : Inport  Port=2
  "    " : Fcn  Expr=-u(1)/2 + u(2)*sqrt(3)/2
  "        " : Fcn  Expr=-u(1)/2 - u(2)*sqrt(3)/2
  Mux3 : Mux  Inputs=2
  a : Outport
  b : Outport  Port=2
  c : Outport  Port=3
  wires:
  alpha/1 -> a/1, Mux3/1
  beta/1 -> Mux3/2
  Mux3/1 -> "    "/1, "        "/1
  "        "/1 -> c/1
  "    "/1 -> b/1

== system AC_FOC_PMSM_Developing_Rev_5_2022b/Simplified_Speed_Q_FLC_D_PID1/Inverse Park-Clarke3/Inverse Park ==
  Id : Inport
  Iq : Inport  Port=2
  theta : Inport  Port=3
  " " : Fcn  Expr=cos(u(3))*u(1)-sin(u(3))*u(2)
  "  " : Fcn  Expr=sin(u(3))*u(1)+cos(u(3))*u(2)
  Mux : Mux  Inputs=3
  alpha : Outport
  beta : Outport  Port=2
  wires:
  Mux/1 -> " "/1, "  "/1
  theta/1 -> Mux/3
  Id/1 -> Mux/1
  Iq/1 -> Mux/2
  " "/1 -> alpha/1
  "  "/1 -> beta/1

== system AC_FOC_PMSM_Developing_Rev_5_2022b/Simplified_Speed_Q_FLC_D_PID1/Subsystem4/Subsystem1 ==
  Constant : Constant
  Constant1 : Constant
  Gain : Gain  Gain=2*10000
  Gain1 : Gain  Gain=2
  Integrator : Integrator
  Pulse Generator : DiscretePulseGenerator  PulseType=Time based  Amplitude=2  Period=1/10000  PulseWidth=50
  Sum3 : Sum  Inputs=|+-
  Sum4 : Sum  Inputs=|+-
  triangle_pulse : Outport
  wires:
  Integrator/1 -> Gain/1
  Sum4/1 -> triangle_pulse/1
  Sum3/1 -> Integrator/1
  Gain/1 -> Gain1/1
  Constant1/1 -> Sum4/2
  Constant/1 -> Sum3/2
  Gain1/1 -> Sum4/1
  Pulse Generator/1 -> Sum3/1

== system AC_FOC_PMSM_Developing_Rev_5_2022b/Speed_Q_FLC_D_PID/Inverse Park-Clarke3/Inverse Clarke ==
  alpha : Inport
  beta : Inport  Port=2
  "    " : Fcn  Expr=-u(1)/2 + u(2)*sqrt(3)/2
  "        " : Fcn  Expr=-u(1)/2 - u(2)*sqrt(3)/2
  Mux3 : Mux  Inputs=2
  a : Outport
  b : Outport  Port=2
  c : Outport  Port=3
  wires:
  alpha/1 -> a/1, Mux3/1
  beta/1 -> Mux3/2
  Mux3/1 -> "    "/1, "        "/1
  "        "/1 -> c/1
  "    "/1 -> b/1

== system AC_FOC_PMSM_Developing_Rev_5_2022b/Speed_Q_FLC_D_PID/Inverse Park-Clarke3/Inverse Park ==
  Id : Inport
  Iq : Inport  Port=2
  theta : Inport  Port=3
  " " : Fcn  Expr=cos(u(3))*u(1)-sin(u(3))*u(2)
  "  " : Fcn  Expr=sin(u(3))*u(1)+cos(u(3))*u(2)
  Mux : Mux  Inputs=3
  alpha : Outport
  beta : Outport  Port=2
  wires:
  Mux/1 -> " "/1, "  "/1
  theta/1 -> Mux/3
  Id/1 -> Mux/1
  Iq/1 -> Mux/2
  " "/1 -> alpha/1
  "  "/1 -> beta/1

== system AC_FOC_PMSM_Developing_Rev_5_2022b/Speed_Q_FLC_D_PID/Subsystem4/Subsystem1 ==
  Constant : Constant
  Constant1 : Constant
  Gain : Gain  Gain=2*10000
  Gain1 : Gain  Gain=2
  Integrator : Integrator
  Pulse Generator : DiscretePulseGenerator  PulseType=Time based  Amplitude=2  Period=1/10000  PulseWidth=50
  Sum3 : Sum  Inputs=|+-
  Sum4 : Sum  Inputs=|+-
  triangle_pulse : Outport
  wires:
  Integrator/1 -> Gain/1
  Sum4/1 -> triangle_pulse/1
  Sum3/1 -> Integrator/1
  Gain/1 -> Gain1/1
  Constant1/1 -> Sum4/2
  Constant/1 -> Sum3/2
  Gain1/1 -> Sum4/1
  Pulse Generator/1 -> Sum3/1
